simulink model "MoTran"  (R2023b)
settings: Solver=VariableStepAuto  StartTime=0.0  StopTime=20  RelTol=1e-3
values from neighbouring files (symbols this model uses):
  b1 = 1000    [MoTra.m]    (also in MoTran.mat)
  k1 = 16182    [MoTra.m]    (also in MoTran.mat)
  k2 = 19000    [MoTra.m]    (also in MoTran.mat)
  m1 = 290    [MoTra.m]    (also in MoTran.mat)
  m2 = 59    [MoTra.m]    (also in MoTran.mat)

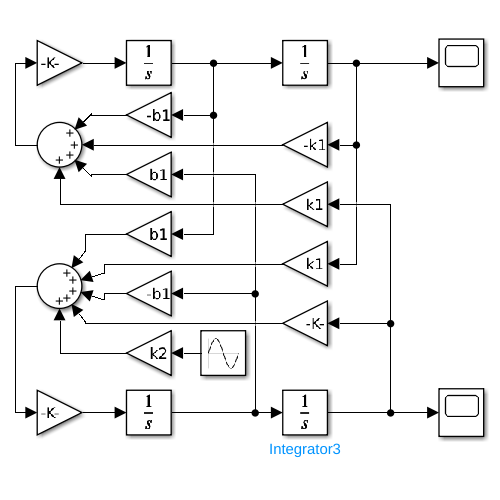
[thumbnail: Simulink's stored preview of the top-level diagram]
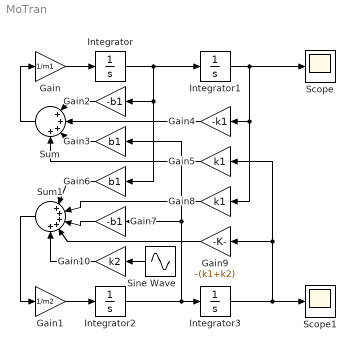
== system MoTran ==
  Gain : Gain  Gain=1/m1
  Gain1 : Gain  Gain=1/m2
  Gain10 : Gain  Gain=k2
  Gain2 : Gain  Gain=-b1
  Gain3 : Gain  Gain=b1
  Gain4 : Gain  Gain=-k1
  Gain5 : Gain  Gain=k1
  Gain6 : Gain  Gain=b1
  Gain7 : Gain  Gain=-b1
  Gain8 : Gain  Gain=k1
  Gain9 : Gain  Gain=-(k1+k2)
  Integrator{,1..3} (4 alike) : Integrator
  Scope : Scope
  Scope1 : Scope
  Sine Wave : Sin  Amplitude=0.05  Frequency=0.5*pi  SampleTime=0
  Sum : Sum  Inputs=|++++
  Sum1 : Sum  Inputs=|+++++
  wires:
  Integrator/1 -> Gain6/1, Gain2/1, Integrator1/1
  Integrator1/1 -> Gain4/1, Gain8/1, Scope/1
  Gain/1 -> Integrator/1
  Integrator2/1 -> Gain7/1, Gain3/1, Integrator3/1
  Gain1/1 -> Integrator2/1
  Integrator3/1 -> Gain9/1, Gain5/1, Scope1/1
  Gain4/1 -> Sum/2
  Gain5/1 -> Sum/4
  Gain2/1 -> Sum/1
  Gain3/1 -> Sum/3
  Sum/1 -> Gain/1
  Gain8/1 -> Sum1/2
  Gain9/1 -> Sum1/4
  Sine Wave/1 -> Gain10/1
  Sum1/1 -> Gain1/1
  Gain10/1 -> Sum1/5
  Gain7/1 -> Sum1/3
  Gain6/1 -> Sum1/1
